simulink model "aero_radmod_dsp"  (Simulink 6.0)
settings: Solver=FixedStepDiscrete  SolverMode=SingleTasking  StartTime=0.0  StopTime=100  MaxStep=0.1  RelTol=1e-3  AbsTol=1e-6
PreLoadFcn:
  | aero_raddat;
StopFcn:
  | aero_radplot;
undefined symbols (not defined in the file or in its folder): deltat, DiscIntNeverNeededParam, g, Speed, tauc, tauT
libraries: dspmtrx3 x9, simulink x7, dspsrcs4 x3, dspsigops x2, dspsolvers x1
CloseFcn:
  | h=findobj('type','figure');if ~isempty(h);close(h);end
settings Model: CovMetricSettings=d  Creator=raberg  LastModifiedBy=hshivaku  ExtModeTrigMode=oneshot  ExtModeArmWhenConnect=off  ExtModeAutoUpdateStatusClock=off
settings DataIOCC: LimitDataPoints=off  SaveOutput=off  SaveTime=off  TimeSaveName=t_sim  SignalLoggingName=sigsOut
settings OptimizationCC: InlineInvariantSignals=off
settings DebuggingCC: CheckExecutionContextPreStartOutputMsg=on  CheckExecutionContextRuntimeOutputMsg=on  SolverPrmCheckMsg=none
settings HardwareCC: TargetUnknown=on
settings RTWCC: GenerateReport=on
settings SFSimCC: SFSimApplyToAllLibs=on  SFSimBuildMode=Incremental

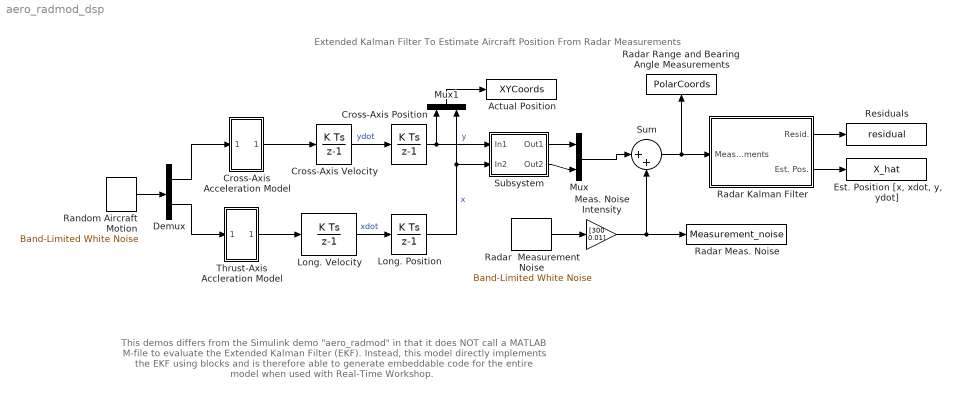
== system aero_radmod_dsp ==
  note: Extended Kalman Filter To Estimate Aircraft Position From Radar Measurements
  note: This demos differs from the Simulink demo "aero_radmod"
      | in that it does NOT call a MATLAB M-file to evaluate the
      | Extended Kalman Filter (EKF).
      |
      | Instead, this model directly implements the EKF using
      | blocks and is therefore able to generate embeddable code
      | for the entire model when used with Real-Time Workshop.
  Actual Position : ToWorkspace  VariableName=XYCoords  SaveFormat=Array
  Cross-Axis Acceleration Model : Subsystem  PropExecContextAcrossSSBoundary=on
  Cross-Axis Position : DiscreteIntegrator  SampleTime=-1  ICPrevOutput=DiscIntNeverNeededParam  ICPrevScaledInput=DiscIntNeverNeededParam
  Cross-Axis Velocity : DiscreteIntegrator  SampleTime=-1  ICPrevOutput=DiscIntNeverNeededParam  ICPrevScaledInput=DiscIntNeverNeededParam
  Demux : Demux  Outputs=2
  "Est. Position [x, xdot, y, ydot]" : ToWorkspace  VariableName=X_hat  SampleTime=-1  SaveFormat=Array
  Long. Position : DiscreteIntegrator  SampleTime=-1  ICPrevOutput=DiscIntNeverNeededParam  ICPrevScaledInput=DiscIntNeverNeededParam
  Long. Velocity : DiscreteIntegrator  InitialCondition=Speed  SampleTime=.1  ICPrevOutput=DiscIntNeverNeededParam  ICPrevScaledInput=DiscIntNeverNeededParam
  Meas. Noise Intensity : Gain  Gain=[300 0.01]  SaturateOnIntegerOverflow=on
  Mux : Mux  Inputs=2
  Mux1 : Mux  Orientation=up  Inputs=2
  Radar Kalman Filter : Subsystem  PropExecContextAcrossSSBoundary=on
  Radar  Measurement Noise : simulink/Sources/Band-Limited White Noise  Cov=[1 1]  Ts=0.1  seed=[52341 62341]
  Radar Meas. Noise : ToWorkspace  VariableName=Measurement_noise  SaveFormat=Array
  Radar Range and Bearing  Angle Measurements : ToWorkspace  VariableName=PolarCoords  SampleTime=-1  SaveFormat=Array
      settings: Orientation=up
  Random Aircraft Motion : simulink/Sources/Band-Limited White Noise  Cov=[0.001 .001]  Ts=0.1  seed=[58413 74925]
  Residuals : ToWorkspace  VariableName=residual  SampleTime=-1  SaveFormat=Array
  Subsystem : Subsystem  PropExecContextAcrossSSBoundary=on
      mask Display: disp('Cartesian\nto Polar')
  Sum : Sum  Inputs=|++  SaturateOnIntegerOverflow=on  InputSameDT=on
  Thrust-Axis Accleration Model : Subsystem  PropExecContextAcrossSSBoundary=on
  wires:
  Long. Position/1 -> Mux1/2, Subsystem/2(In2)  "x"
  Subsystem/2(Out2) -> Mux/2
  Subsystem/1(Out1) -> Mux/1
  Mux/1 -> Sum/1
  Sum/1 -> Radar Range and Bearing  Angle Measurements/1, Radar Kalman Filter/1(Measurements)
  Cross-Axis Position/1 -> Mux1/1, Subsystem/1(In1)  "y"
  Cross-Axis Acceleration Model/1(Out) -> Cross-Axis Velocity/1
  Cross-Axis Velocity/1 -> Cross-Axis Position/1  "ydot"
  Long. Velocity/1 -> Long. Position/1  "xdot"
  Thrust-Axis Accleration Model/1(Accleration) -> Long. Velocity/1
  Radar Kalman Filter/1(Resid.) -> Residuals/1
  Demux/1 -> Cross-Axis Acceleration Model/1(Inport)
  Demux/2 -> Thrust-Axis Accleration Model/1(Force)
  Meas. Noise Intensity/1 -> Radar Meas. Noise/1, Sum/2
  Mux1/1 -> Actual Position/1
  Radar Kalman Filter/2(Est. Pos.) -> "Est. Position [x, xdot, y, ydot]"/1
  Radar  Measurement Noise/1 -> Meas. Noise Intensity/1
  Random Aircraft Motion/1 -> Demux/1

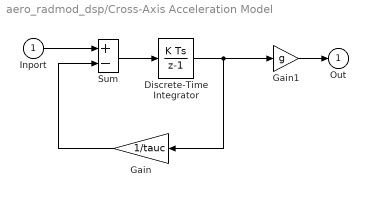
== system aero_radmod_dsp/Cross-Axis Acceleration Model ==
  Inport : Inport  LatchInput=off
  Discrete-Time Integrator : DiscreteIntegrator  SampleTime=-1  ICPrevOutput=DiscIntNeverNeededParam  ICPrevScaledInput=DiscIntNeverNeededParam
  Gain : Gain  Orientation=left  Gain=1/tauc  SaturateOnIntegerOverflow=on
  Gain1 : Gain  Gain=g  SaturateOnIntegerOverflow=on
  Sum : Sum  Inputs=+-  SaturateOnIntegerOverflow=on  InputSameDT=on
  Out : Outport  InitialOutput=0
  wires:
  Sum/1 -> Discrete-Time Integrator/1
  Gain1/1 -> Out/1
  Discrete-Time Integrator/1 -> Gain/1, Gain1/1
  Gain/1 -> Sum/2
  Inport/1 -> Sum/1

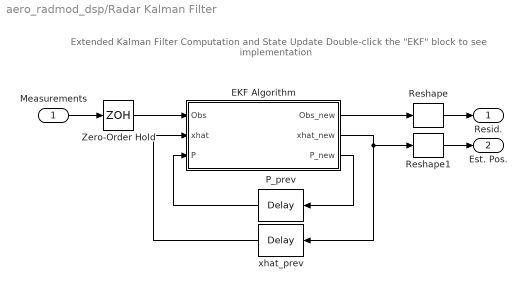
== system aero_radmod_dsp/Radar Kalman Filter ==
  note: Extended Kalman Filter
      | Computation and State Update
      |
      | Double-click the "EKF" block to see implementation
  Measurements : Inport  LatchInput=off
  EKF Algorithm : Subsystem  PropExecContextAcrossSSBoundary=on
      mask Display: disp('EKF')
  P_prev : dspsigops/Delay  Orientation=left  dly_unit=Samples  delay=1  ic_detail=off  dif_ic_for_ch=off  dif_ic_for_dly=off  ic=0  reset_popup=None
  Reshape : simulink/Math Operations/Reshape  OutputDimensionality=1-D array  OutputDimensions=[1,1]
  Reshape1 : simulink/Math Operations/Reshape  OutputDimensionality=1-D array  OutputDimensions=[1,1]
  Zero-Order Hold : ZeroOrderHold  SampleTime=deltat
  xhat_prev : dspsigops/Delay  Orientation=left  dly_unit=Samples  delay=1  ic_detail=on  dif_ic_for_ch=on  dif_ic_for_dly=off  ic=[0.001, 0.01, 0.001, 400]  reset_popup=None
  Resid. : Outport  InitialOutput=0
  Est. Pos. : Outport  Port=2  InitialOutput=0
  wires:
  Measurements/1 -> Zero-Order Hold/1
  Zero-Order Hold/1 -> EKF Algorithm/1(Obs)
  EKF Algorithm/3(P_new) -> P_prev/1
  EKF Algorithm/2(xhat_new) -> xhat_prev/1, Reshape1/1
  EKF Algorithm/1(Obs_new) -> Reshape/1
  Reshape/1 -> Resid./1
  Reshape1/1 -> Est. Pos./1
  P_prev/1 -> EKF Algorithm/3(P)
  xhat_prev/1 -> EKF Algorithm/2(xhat)

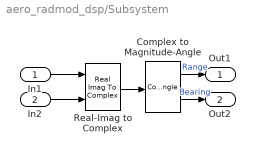
== system aero_radmod_dsp/Subsystem ==
  In1 : Inport  LatchInput=off
  In2 : Inport  Port=2  LatchInput=off
  Complex to Magnitude-Angle : ComplexToMagnitudeAngle
  Real-Imag to Complex : RealImagToComplex
  Out1 : Outport
  Out2 : Outport  Port=2
  wires:
  Real-Imag to Complex/1 -> Complex to Magnitude-Angle/1
  In1/1 -> Real-Imag to Complex/1
  In2/1 -> Real-Imag to Complex/2
  Complex to Magnitude-Angle/1 -> Out1/1  "Range"
  Complex to Magnitude-Angle/2 -> Out2/1  "Bearing"

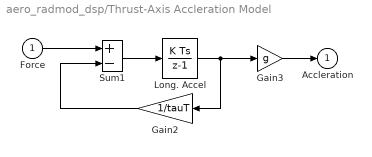
== system aero_radmod_dsp/Thrust-Axis Accleration Model ==
  Force : Inport  LatchInput=off
  Gain2 : Gain  Orientation=left  Gain=1/tauT  SaturateOnIntegerOverflow=on
  Gain3 : Gain  Gain=g  SaturateOnIntegerOverflow=on
  Long. Accel : DiscreteIntegrator  SampleTime=-1  ICPrevOutput=DiscIntNeverNeededParam  ICPrevScaledInput=DiscIntNeverNeededParam
  Sum1 : Sum  Inputs=+-  SaturateOnIntegerOverflow=on  InputSameDT=on
  Accleration : Outport  InitialOutput=0
  wires:
  Gain3/1 -> Accleration/1
  Sum1/1 -> Long. Accel/1
  Long. Accel/1 -> Gain2/1, Gain3/1
  Gain2/1 -> Sum1/2
  Force/1 -> Sum1/1

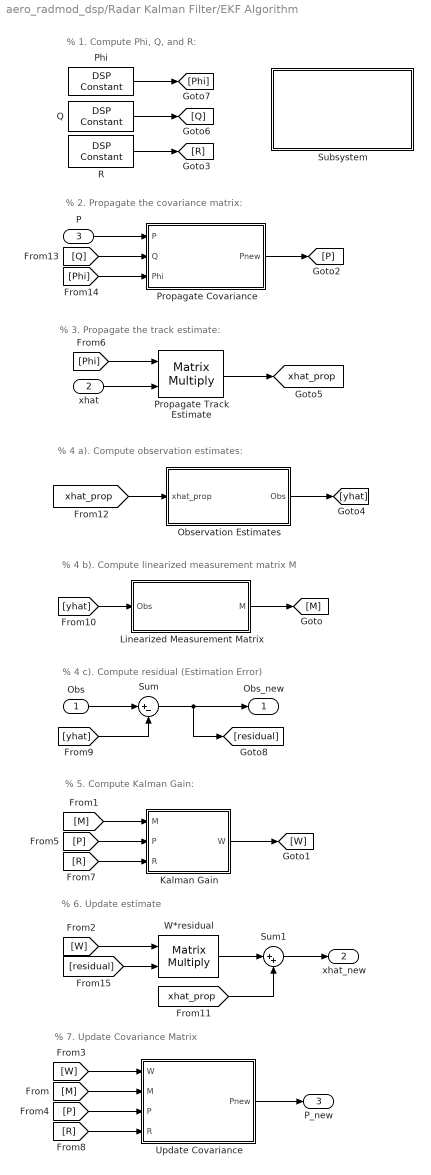
== system aero_radmod_dsp/Radar Kalman Filter/EKF Algorithm ==
  note: % 1. Compute Phi, Q, and R:
  note: % 2. Propagate the covariance matrix:
  note: % 3. Propagate the track estimate:
  note: % 4 a). Compute observation estimates:
  note: % 4 b). Compute linearized measurement matrix M
  note: % 4 c). Compute residual (Estimation Error)
  note: % 5. Compute Kalman Gain:
  note: % 6. Update estimate
  note: % 7. Update Covariance Matrix
  Obs : Inport  LatchInput=off
  xhat : Inport  Port=2  PortDimensions=[4 1]  LatchInput=off
  P : Inport  Port=3  LatchInput=off
  Kalman Gain : Subsystem  PropExecContextAcrossSSBoundary=on
      mask Display: disp('Kalman\nGain')
  Linearized Measurement Matrix : Subsystem  PropExecContextAcrossSSBoundary=on
      mask Display: disp('Linearized\nMeasurement\nMatrix')
  Observation Estimates : Subsystem  PropExecContextAcrossSSBoundary=on
      mask Display: disp('Observation\n\nEstimates')
  Phi : dspsrcs4/DSP Constant  Value=single([1 deltat 0 0; 0 1 0 0 ; 0 0 1 deltat; 0 0 0 1])  SampleMode=Discrete  discreteOutput=Sample-based  continuousOutput=Sample-based  sampTime=deltat  framePeriod=2  dataType=Inherit via back propagation  wordLen=16  udDataType=sfix(16)  fracBitsMode=Best precision  numFracBits=15  InterpretAs1D=-inf  Ts=-inf  FramebasedOutput=-inf
      settings: additionalParams=on
  Propagate Covariance : Subsystem  PropExecContextAcrossSSBoundary=on
      mask Display: disp('Propagate\nCovariance')
  Propagate Track Estimate : dspmtrx3/Matrix Multiply  numInputPorts=2  OptimizationLevel=None
  Q : dspsrcs4/DSP Constant  Value=single(diag([0 .005 0 .005]))  SampleMode=Discrete  discreteOutput=Sample-based  continuousOutput=Sample-based  sampTime=deltat  framePeriod=2  dataType=Inherit via back propagation  wordLen=16  udDataType=sfix(16)  fracBitsMode=Best precision  numFracBits=15  InterpretAs1D=-inf  Ts=-inf  FramebasedOutput=-inf
      settings: additionalParams=on
  R : dspsrcs4/DSP Constant  Value=single(diag([300^2 0.001^2]))  SampleMode=Discrete  discreteOutput=Sample-based  continuousOutput=Sample-based  sampTime=deltat  framePeriod=2  dataType=Inherit via back propagation  wordLen=16  udDataType=sfix(16)  fracBitsMode=Best precision  numFracBits=15  InterpretAs1D=-inf  Ts=-inf  FramebasedOutput=-inf
      settings: additionalParams=on
  Subsystem : Subsystem  PropExecContextAcrossSSBoundary=on
      settings: OpenFcn=edit aero_extkalman
      mask Display:
      | disp('Implementation of\n ...
      | Extended Kalman Filter\n ...
      | closely follows M-file\n ...
      | "aero_extkalman.m"\n\n ...
      | Click here to view M-file.');
  Sum : Sum  Inputs=|+-  SaturateOnIntegerOverflow=on
  Sum1 : Sum  Inputs=|++  SaturateOnIntegerOverflow=on
  Update Covariance : Subsystem  PropExecContextAcrossSSBoundary=on
      mask Display: disp('Update\nCovariance')
  W*residual : dspmtrx3/Matrix Multiply  numInputPorts=2  OptimizationLevel=None
  Obs_new : Outport
  xhat_new : Outport  Port=2
  P_new : Outport  Port=3
  tag scope: xhat_prop=global
  wires:
  P/1 -> Propagate Covariance/1(P)
  [Phi] -> Propagate Track Estimate/1
  [Q] -> Propagate Covariance/2(Q)
  xhat/1 -> Propagate Track Estimate/2
  Propagate Track Estimate/1 -> [xhat_prop]
  Linearized Measurement Matrix/1(M) -> [M]
  [R] -> Kalman Gain/3(R)
  [M] -> Update Covariance/2(M)
  [M] -> Kalman Gain/1(M)
  Kalman Gain/1(W) -> [W]
  [W] -> W*residual/1
  [P] -> Update Covariance/3(P)
  Propagate Covariance/1(Pnew) -> [P]
  [P] -> Kalman Gain/2(P)
  R/1 -> [R]
  [R] -> Update Covariance/4(R)
  Update Covariance/1(Pnew) -> P_new/1
  [yhat] -> Linearized Measurement Matrix/1(Obs)
  [xhat_prop] -> Observation Estimates/1(xhat_prop)
  Q/1 -> [Q]
  [W] -> Update Covariance/1(W)
  Observation Estimates/1(Obs) -> [yhat]
  Phi/1 -> [Phi]
  [Phi] -> Propagate Covariance/3(Phi)
  Sum1/1 -> xhat_new/1
  [residual] -> W*residual/2
  Obs/1 -> Sum/1
  [yhat] -> Sum/2
  W*residual/1 -> Sum1/1
  [xhat_prop] -> Sum1/2
  Sum/1 -> Obs_new/1, [residual]

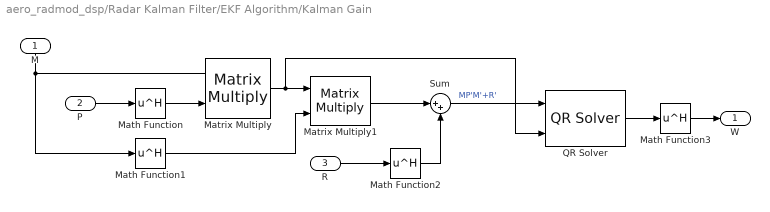
== system aero_radmod_dsp/Radar Kalman Filter/EKF Algorithm/Kalman Gain ==
  M : Inport  Orientation=down  LatchInput=off
  P : Inport  Port=2  LatchInput=off
  R : Inport  Port=3  LatchInput=off
  Math Function{,1..3} (4 alike) : Math  Operator=hermitian  SaturateOnIntegerOverflow=on
  Matrix Multiply : dspmtrx3/Matrix Multiply  numInputPorts=2  OptimizationLevel=None
  Matrix Multiply1 : dspmtrx3/Matrix Multiply  numInputPorts=2  OptimizationLevel=None
  QR Solver : dspsolvers/QR Solver
  Sum : Sum  Inputs=|++  SaturateOnIntegerOverflow=on
  W : Outport
  wires:
  R/1 -> Math Function2/1
  Sum/1 -> QR Solver/1  "MP'M'+R'"
  M/1 -> Matrix Multiply/1, Math Function1/1
  P/1 -> Math Function/1
  Math Function/1 -> Matrix Multiply/2
  Matrix Multiply/1 -> Matrix Multiply1/1, QR Solver/2
  Math Function1/1 -> Matrix Multiply1/2
  Matrix Multiply1/1 -> Sum/1
  Math Function2/1 -> Sum/2
  QR Solver/1 -> Math Function3/1
  Math Function3/1 -> W/1

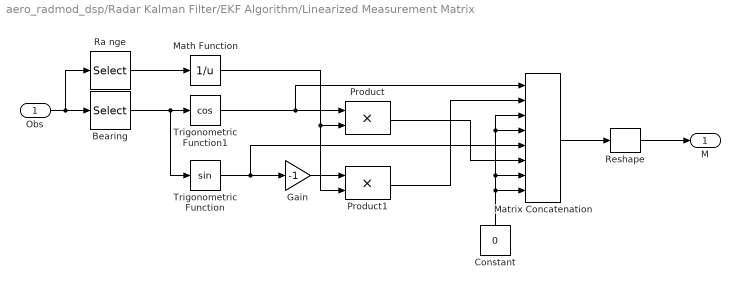
== system aero_radmod_dsp/Radar Kalman Filter/EKF Algorithm/Linearized Measurement Matrix ==
  Obs : Inport  LatchInput=off
  Bearing : Selector  Elements=2  InputPortWidth=2
  Constant : Constant  Orientation=up  Value=0
  Gain : Gain  Gain=-1  SaturateOnIntegerOverflow=on
  Math Function : Math  Operator=reciprocal  SaturateOnIntegerOverflow=on
  Matrix Concatenation : simulink/Math Operations/Matrix Concatenation  numInports=8  catMethod=Vertical
  Product : Product  SaturateOnIntegerOverflow=on
  Product1 : Product  SaturateOnIntegerOverflow=on
  Ra nge : Selector  InputPortWidth=2
  Reshape : simulink/Math Operations/Reshape  OutputDimensionality=Customize  OutputDimensions=[2,4]
  Trigonometric Function : Trigonometry
  Trigonometric Function1 : Trigonometry  Operator=cos
  M : Outport
  wires:
  Obs/1 -> Bearing/1, Ra nge/1
  Bearing/1 -> Trigonometric Function1/1, Trigonometric Function/1
  Ra nge/1 -> Math Function/1
  Trigonometric Function1/1 -> Product/1, Matrix Concatenation/1
  Trigonometric Function/1 -> Gain/1, Matrix Concatenation/5
  Math Function/1 -> Product/2, Product1/2
  Gain/1 -> Product1/1
  Product1/1 -> Matrix Concatenation/2
  Product/1 -> Matrix Concatenation/6
  Matrix Concatenation/1 -> Reshape/1
  Constant/1 -> Matrix Concatenation/8, Matrix Concatenation/7, Matrix Concatenation/4, Matrix Concatenation/3
  Reshape/1 -> M/1

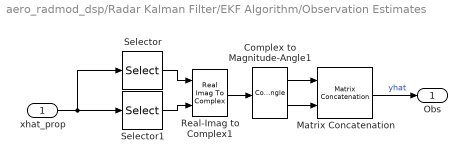
== system aero_radmod_dsp/Radar Kalman Filter/EKF Algorithm/Observation Estimates ==
  xhat_prop : Inport  LatchInput=off
  Complex to Magnitude-Angle1 : ComplexToMagnitudeAngle
  Matrix Concatenation : simulink/Math Operations/Matrix Concatenation  numInports=2  catMethod=Vertical
  Real-Imag to Complex1 : RealImagToComplex
  Selector : Selector  InputPortWidth=4
  Selector1 : Selector  Elements=3  InputPortWidth=4
  Obs : Outport
  wires:
  xhat_prop/1 -> Selector1/1, Selector/1
  Real-Imag to Complex1/1 -> Complex to Magnitude-Angle1/1
  Selector/1 -> Real-Imag to Complex1/1
  Selector1/1 -> Real-Imag to Complex1/2
  Complex to Magnitude-Angle1/1 -> Matrix Concatenation/1
  Complex to Magnitude-Angle1/2 -> Matrix Concatenation/2
  Matrix Concatenation/1 -> Obs/1  "yhat"

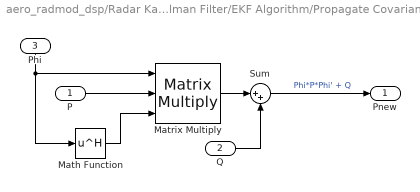
== system aero_radmod_dsp/Radar Kalman Filter/EKF Algorithm/Propagate Covariance ==
  P : Inport  LatchInput=off
  Q : Inport  Port=2  LatchInput=off
  Phi : Inport  Orientation=down  Port=3  LatchInput=off
  Math Function : Math  Operator=hermitian  SaturateOnIntegerOverflow=on
  Matrix Multiply : dspmtrx3/Matrix Multiply  numInputPorts=3  OptimizationLevel=None
  Sum : Sum  Inputs=|++  SaturateOnIntegerOverflow=on
  Pnew : Outport
  wires:
  Math Function/1 -> Matrix Multiply/3
  Matrix Multiply/1 -> Sum/1
  Phi/1 -> Math Function/1, Matrix Multiply/1
  P/1 -> Matrix Multiply/2
  Sum/1 -> Pnew/1  "Phi*P*Phi' + Q"
  Q/1 -> Sum/2

== system aero_radmod_dsp/Radar Kalman Filter/EKF Algorithm/Subsystem ==

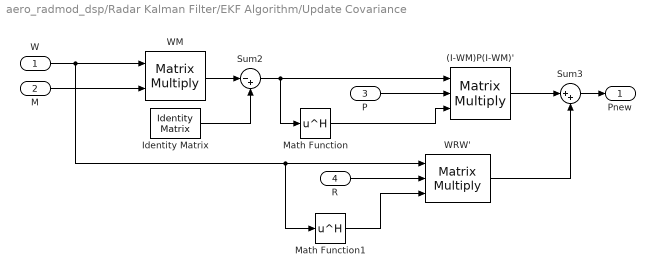
== system aero_radmod_dsp/Radar Kalman Filter/EKF Algorithm/Update Covariance ==
  W : Inport  LatchInput=off
  M : Inport  Port=2  LatchInput=off
  P : Inport  Port=3  LatchInput=off
  R : Inport  Port=4  LatchInput=off
  (I-WM)P(I-WM)' : dspmtrx3/Matrix Multiply  numInputPorts=3  OptimizationLevel=None
  Identity Matrix : dspmtrx3/Identity Matrix  Inherit=off  N=4  Ts=deltat  dataType=Inherit via back propagation  wordLen=16  udDataType=sfix(16)  fracBitsMode=Best precision  numFracBits=15
      settings: additionalParams=on
  Math Function : Math  Operator=hermitian  SaturateOnIntegerOverflow=on
  Math Function1 : Math  Operator=hermitian  SaturateOnIntegerOverflow=on
  Sum2 : Sum  Inputs=|-+  SaturateOnIntegerOverflow=on
  Sum3 : Sum  Inputs=|++  SaturateOnIntegerOverflow=on
  WM : dspmtrx3/Matrix Multiply  numInputPorts=2  OptimizationLevel=None
  WRW' : dspmtrx3/Matrix Multiply  numInputPorts=3  OptimizationLevel=None
  Pnew : Outport
  wires:
  W/1 -> Math Function1/1, WRW'/1, WM/1
  Sum2/1 -> (I-WM)P(I-WM)'/1, Math Function/1
  Math Function/1 -> (I-WM)P(I-WM)'/3
  Math Function1/1 -> WRW'/3
  (I-WM)P(I-WM)'/1 -> Sum3/1
  WRW'/1 -> Sum3/2
  Identity Matrix/1 -> Sum2/2
  WM/1 -> Sum2/1
  M/1 -> WM/2
  P/1 -> (I-WM)P(I-WM)'/2
  Sum3/1 -> Pnew/1
  R/1 -> WRW'/2
